simulink model "heli_q8_d6p2"  (R2018b)
settings: Solver=ode1  StartTime=0.0  StopTime=inf  FixedStep=0.002  RelTol=1e-3  EnableMultiTasking=on
PostLoadFcn:
  | qc_set_target_type(getConfigSet(bdroot, 'QUARC Default Target Configuration'));
values from neighbouring files (symbols this model uses):
  A_d = sys_disc.A    [Dag6.m]    (also in Dag6p2.m)
  B_d = sys_disc.B    [Dag6.m]    (also in Dag6p2.m)
  C_d = sys_disc.C    [Dag6.m]    (also in Dag6p2.m)
  Q_d = diag([0.0001 0.001 0.001 0.001 0.0001 0.0001])    [Dag6.m]    (also in Dag6p2.m = diag([Q_d_p Q_d_pdot Q_d_e Q_d_edot Q_d_l Q_d_ldot]))
  R_d = R_d(1:5, 1:5)    [Dag6.m]    (also in Dag6p2.m = cov(Noise_flying_vals_no_time.', 'omitrows'))
undefined symbols (not defined in the file or in its folder): HIL
libraries: quarc_library x1
settings Model: SimulationMode=external  ExtModeTrigDuration=5000  Creator=Rchan  LastModifiedBy=patricknitschke
settings SolverCC: PositivePriorityOrder=on
settings DataIOCC: LimitDataPoints=on  SaveFormat=Array  SignalLoggingSaveFormat=ModelDataLogs
settings OptimizationCC: ExpressionDepthLimit=2147483647  InitFltsAndDblsToZero=on  LifeSpan=inf
settings DebuggingCC: SaveWithParameterizedLinksMsg=none  UnderspecifiedInitializationDetection=Classic  MergeDetectMultiDrivingBlocksExec=none  SolverPrmCheckMsg=warning  MultiTaskDSMMsg=warning  MultiTaskCondExecSysMsg=none  FcnCallInpInsideContextMsg=warning  AllowSymbolicDim=off  StateNameClashWarn=warning  SFUnexpectedBacktrackingDiag=warning  SFNoUnconditionalDefaultTransitionDiag=warning  SFExecutionAtInitializationDiag=none
settings HardwareCC: ProdBitPerPointer=32  ProdBitPerSizeT=32  ProdBitPerPtrDiffT=32  ProdLargestAtomicFloat=None  ProdIntDivRoundTo=Undefined  ProdEndianess=Unspecified  ProdWordSize=32  ProdHWDeviceType=32-bit Generic
settings ModelReferenceCC: PropagateSignalLabelsOutOfModel=off
settings SFSimCC: SimUseLocalCustomCode=off
settings RTWCC: SystemTargetFile=quarc_win64.tlc  TemplateMakefile=quarc_default_tmf  Description=QUARC Win64 Target  RTWUseLocalCustomCode=off
settings CodeAppCC: StateflowObjectComments=on
settings STFCustomTargetCC: TargetPreCompLibLocation=C:\PROGRA~3\QUARC\lib\2015b\win64\release  ConcurrentExecutionCompliant=on  GeneratePreprocessorConditionals=Disable all  CPPClassGenCompliant=on  GRTInterface=on  SystemTargetFile=quarc_win64.tlc
settings GRTTargetCC: TargetPreCompLibLocation=C:\PROGRA~3\QUARC\lib\2015b\win64\release  TargetLangStandard=C89/C90 (ANSI)  ParMdlRefBuildCompliant=off  CompOptLevelCompliant=off  GeneratePreprocessorConditionals=Disable all  CombineOutputUpdateFcns=off  MatFileLogging=off  GRTInterface=on  UseToolchainInfoCompliant=off  ExtMode=on  ExtModeMexFile=quarc_comm
settings ConfigComp: CovMetricSettings=dw  CovHtmlReporting=on  CovSaveCumulativeToWorkspaceVar=on  CovSaveSingleToWorkspaceVar=on  CovExternalEMLEnable=off  CovSFcnEnable=off

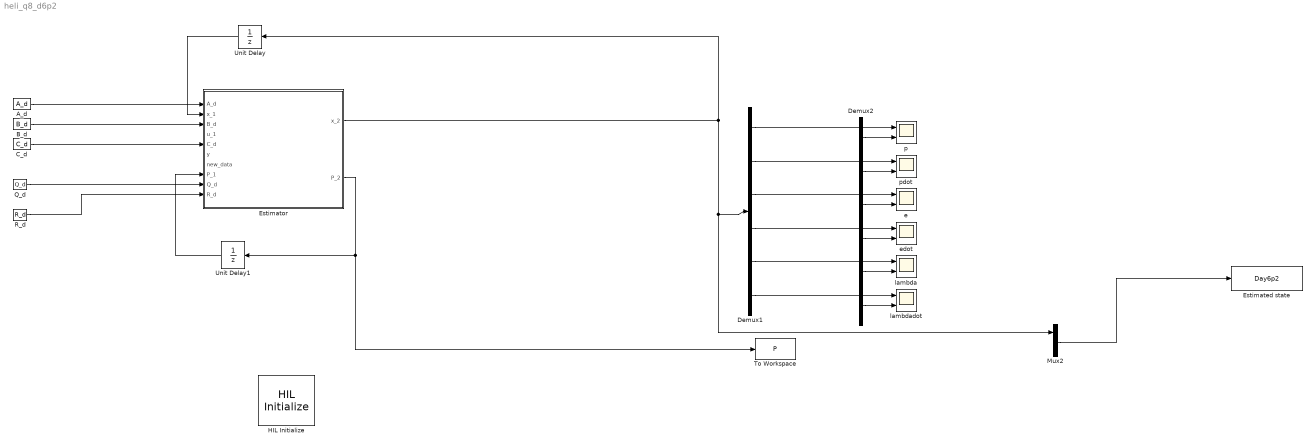
== system heli_q8_d6p2 ==
  A_d : Constant  Value=A_d  VectorParams1D=off  SampleTime=0.002
  B_d : Constant  Value=B_d  VectorParams1D=off  SampleTime=0.002
  C_d : Constant  Value=C_d  VectorParams1D=off  SampleTime=0.002
  Demux1 : Demux  Outputs=6
  Demux2 : Demux  Outputs=6
  Estimated state : ToFile  Filename=Day6p2
  Estimator : MATLAB Function  TreatAsAtomicUnit=on
  HIL Initialize : quarc_library/Data Acquisition/Generic/Configuration/HIL Initialize  Priority=-99  object_name=HIL-1  board_type=q8_usb  board_number=0  board_options=update_rate=normal;decimation=1  exclusive=off  active=off  hardware_clocks=[0:2]  clock_modes=[]  initial_clock_frequencies=[]  set_clock_params_at_start=off  set_clock_params_at_switch_in=off  set_clock_frequencies_at_start=off  set_clock_frequencies_at_switch_in=off  analog_input_channels=[0:7]  analog_input_maximums=10  analog_input_minimums=-10  set_analog_input_params_at_start=on  set_analog_input_params_at_switch_in=off  analog_output_channels=[0:7]  analog_output_maximums=10  analog_output_minimums=-10  initial_analog_outputs=[0]  final_analog_outputs=[0]  watchdog_analog_outputs=0  set_analog_output_params_at_start=on  set_analog_output_params_at_switch_in=off  set_analog_outputs_at_start=on  set_analog_outputs_at_switch_in=off  set_analog_outputs_at_terminate=on  set_analog_outputs_at_switch_out=off  set_analog_outputs_on_watchdog=off  digital_input_channels=[]  digital_output_channels=[]  digital_output_configuration=[]  initial_digital_outputs=[1]  final_digital_outputs=[1]  watchdog_digital_outputs=[1]  set_digital_output_params_at_start=off  set_digital_output_params_at_switch_in=off  set_digital_outputs_at_start=on  set_digital_outputs_at_switch_in=off  set_digital_outputs_at_terminate=on  set_digital_outputs_at_switch_out=off  set_digital_outputs_on_watchdog=off  encoder_channels=[0:7]  quadrature=[4]  encoder_filter_frequency=[]  initial_encoder_counts=[0]  set_encoder_params_at_start=on  set_encoder_params_at_switch_in=off  set_encoder_counts_at_start=on  set_encoder_counts_at_switch_in=off  pwm_channels=[0:7]  pwm_modes=0  pwm_frequency=99.532799999999995e6/4095  pwm_configuration=[0]  pwm_alignment=[0]  pwm_polarity=[1]  pwm_leading_deadband=[0]  pwm_trailing_deadband=[0]  initial_pwm_outputs=[0]  final_pwm_outputs=[0]  watchdog_pwm_outputs=[0]  set_pwm_params_at_start=on  set_pwm_params_at_switch_in=off  set_pwm_outputs_at_start=on  set_pwm_outputs_at_switch_in=off  set_pwm_outputs_at_terminate=on  set_pwm_outputs_at_switch_out=off  set_pwm_outputs_on_watchdog=off  other_output_channels=[]  initial_other_outputs=[]  final_other_outputs=[]  watchdog_other_outputs=[]  set_other_outputs_at_start=off  set_other_outputs_at_switch_in=off  set_other_outputs_at_terminate=off  set_other_outputs_at_switch_out=off  set_other_outputs_on_watchdog=off
  Mux2 : Mux  Inputs=2
  Q_d : Constant  Value=Q_d  VectorParams1D=off  SampleTime=0.002
  R_d : Constant  Value=R_d  VectorParams1D=off  SampleTime=0.002
  To Workspace : ToWorkspace  VariableName=P  SaveFormat=Structure With Time  SampleTime=-1
  Unit Delay : UnitDelay  InitialCondition=[0;0;-0.55;0;0;0]  SampleTime=-1
  Unit Delay1 : UnitDelay  InitialCondition=[0 0 0 0 0 0;0 0 0 0 0 0;0 0 0 0 0 0;0 0 0 0 0 0;0 0 0 0 0 0;0 0 0 0 0 0]  SampleTime=-1
  e : Scope  NumInputPorts=2
  edot : Scope  NumInputPorts=2
  lambda : Scope  NumInputPorts=2
  lambdadot : Scope  NumInputPorts=2
  p : Scope  NumInputPorts=2
  pdot : Scope  NumInputPorts=2
  wires:
  ? -> ?
  Unit Delay/1 -> Estimator/2(x_1)
  Estimator/1(x_2) -> Demux1/1, Mux2/1, Unit Delay/1
  A_d/1 -> Estimator/1(A_d)
  B_d/1 -> Estimator/3(B_d)
  Demux1/1 -> p/1
  Demux1/2 -> pdot/1
  Demux1/3 -> e/1
  Demux1/4 -> edot/1
  Demux1/5 -> lambda/1
  Demux1/6 -> lambdadot/1
  Demux2/6 -> lambdadot/2
  Demux2/5 -> lambda/2
  Demux2/4 -> edot/2
  Demux2/3 -> e/2
  Demux2/2 -> pdot/2
  Demux2/1 -> p/2
  Mux2/1 -> Estimated state/1
  Estimator/2(P_2) -> Unit Delay1/1, To Workspace/1
  Unit Delay1/1 -> Estimator/8(P_1)
  Q_d/1 -> Estimator/9(Q_d)
  C_d/1 -> Estimator/5(C_d)
  R_d/1 -> Estimator/10(R_d)

== matlab function heli_q8_d6p2/Estimator ==
  data: A_d input; x_1 input; B_d input; u_1 input; C_d input; y input; new_data input; x_2 output; P_1 input; P_2 output; Q_d input; R_d input
function [x_2, P_2] = fcn(A_d, x_1, B_d, u_1, C_d, y, new_data, P_1, Q_d, R_d)
%#codegen
I = eye(6);
K = P_1*(C_d.')*(C_d*P_1*(C_d.')+R_d)^-1;
if new_data
    x_hat = (I - K*C_d)*x_1 + K*y;
    P_hat = (I - K*C_d)*P_1*((I-K*C_d).') + K*R_d*(K.');
else
    x_hat = x_1;
    P_hat = P_1;
end
P_2 = A_d*P_hat*(A_d.') + Q_d;
x_2 = A_d*x_hat + B_d*u_1;
